simulink subsystem "ReferenceInputs"  (R2026a)
settings: Solver=VariableStepAuto
undefined symbols (not defined in the file): SimPar
libraries: BezierLib x1
settings Model: Creator=tbritton  LastModifiedBy=pkmas

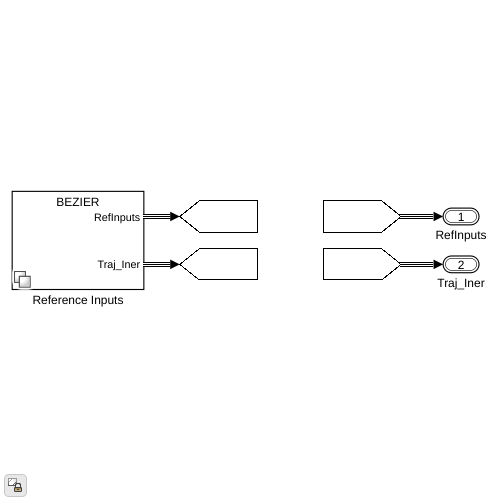
[thumbnail: Simulink's stored preview of the top-level diagram]
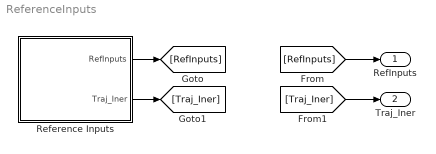
== system ReferenceInputs ==
  Reference Inputs : Subsystem  Variant=on
  RefInputs : Outport  OutDataTypeStr=Bus: BUS_REF_INPUT  VectorParamsAs1DForOutWhenUnconnected=off
  Traj_Iner : Outport  Port=2  OutDataTypeStr=Bus: BUS_REF_INPUT_INER  VectorParamsAs1DForOutWhenUnconnected=off
  wires:
  [RefInputs] -> RefInputs/1
  Reference Inputs/1(RefInputs) -> [RefInputs]
  Reference Inputs/2(Traj_Iner) -> [Traj_Iner]
  [Traj_Iner] -> Traj_Iner/1

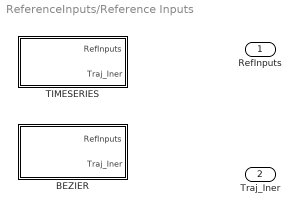
== system ReferenceInputs/Reference Inputs ==
  BEZIER : Subsystem  VariantControl=GVS_REFINPUT_TYPE_BEZIER
  TIMESERIES : Subsystem  VariantControl=GVS_REFINPUT_TYPE_TIMESERIES
  RefInputs : Outport  OutDataTypeStr=Bus: BUS_REF_INPUT  VectorParamsAs1DForOutWhenUnconnected=off
  Traj_Iner : Outport  Port=2  OutDataTypeStr=Bus: BUS_REF_INPUT_INER

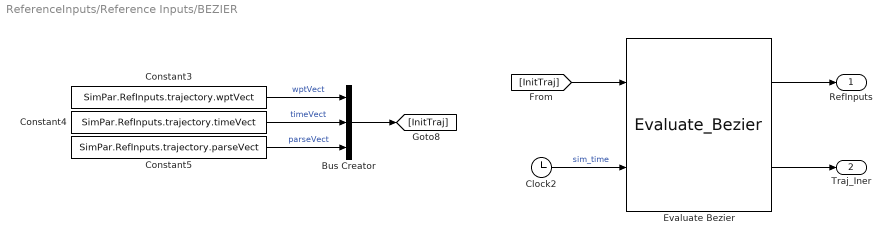
== system ReferenceInputs/Reference Inputs/BEZIER ==
  Bus Creator : BusCreator  Inputs=3
  Clock2 : Clock
  Constant3 : Constant  Value=SimPar.RefInputs.trajectory.wptVect
  Constant4 : Constant  Value=SimPar.RefInputs.trajectory.timeVect
  Constant5 : Constant  Value=SimPar.RefInputs.trajectory.parseVect
  Evaluate Bezier : BezierLib/Evaluate_Bezier  tlen_max=1
  RefInputs : Outport
  Traj_Iner : Outport  Port=2
  wires:
  Bus Creator/1 -> [InitTraj]
  Constant5/1 -> Bus Creator/3  "parseVect"
  Constant4/1 -> Bus Creator/2  "timeVect"
  Constant3/1 -> Bus Creator/1  "wptVect"
  Evaluate Bezier/2 -> Traj_Iner/1
  Evaluate Bezier/1 -> RefInputs/1
  Clock2/1 -> Evaluate Bezier/2  "sim_time"
  [InitTraj] -> Evaluate Bezier/1

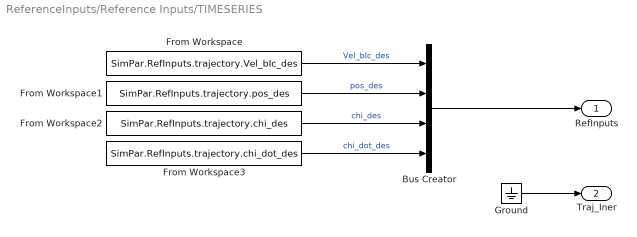
== system ReferenceInputs/Reference Inputs/TIMESERIES ==
  Bus Creator : BusCreator  Inputs=4
  From Workspace : FromWorkspace  VariableName=SimPar.RefInputs.trajectory.Vel_bIc_des  OutputAfterFinalValue=Holding final value
  From Workspace1 : FromWorkspace  VariableName=SimPar.RefInputs.trajectory.pos_des  OutputAfterFinalValue=Holding final value
  From Workspace2 : FromWorkspace  VariableName=SimPar.RefInputs.trajectory.chi_des  OutputAfterFinalValue=Holding final value
  From Workspace3 : FromWorkspace  VariableName=SimPar.RefInputs.trajectory.chi_dot_des  OutputAfterFinalValue=Holding final value
  Ground : Ground
  RefInputs : Outport
  Traj_Iner : Outport  Port=2
  wires:
  Bus Creator/1 -> RefInputs/1
  From Workspace3/1 -> Bus Creator/4  "chi_dot_des"
  From Workspace2/1 -> Bus Creator/3  "chi_des"
  From Workspace1/1 -> Bus Creator/2  "pos_des"
  From Workspace/1 -> Bus Creator/1  "Vel_bIc_des"
  Ground/1 -> Traj_Iner/1
